simulink model "mpc_cstr_multiple"  (R2025a)
settings: Solver=ode45  StartTime=0  StopTime=60  RelTol=1e-3  EnableMultiTasking=on
values from neighbouring files (symbols this model uses):
  mpcobj = mpc(plant,Ts)    [mpccstr.m]
undefined symbols (not defined in the file or in its folder): CSTR_Setpoints
libraries: mpclib x1
settings Model: Creator=The MathWorks, Inc.  LastModifiedBy=The MathWorks, Inc.
settings SolverCC: AlgebraicLoopSolver=TrustRegion
settings DataIOCC: InitialState=[311.261171037073;8.57000022595505;298.146416805263]  SaveFormat=StructureWithTime  SaveOutput=off  SaveState=on  SignalLogging=off  SaveTime=off  ReturnWorkspaceOutputs=off  SignalLoggingName=logsOut
settings OptimizationCC: BooleanDataType=off  DefaultParameterBehavior=Inlined  InlineInvariantSignals=on  BufferReuse=off  ExpressionDepthLimit=2147483647.0  InitFltsAndDblsToZero=on  EfficientMapNaN2IntZero=off  LifeSpan=inf
settings DebuggingCC: AlgebraicLoopMsg=none  SaveWithParameterizedLinksMsg=none  UnderspecifiedInitializationDetection=Classic  MergeDetectMultiDrivingBlocksExec=none  CheckExecutionContextPreStartOutputMsg=on  SignalResolutionControl=TryResolveAllWithWarning  MultiTaskDSMMsg=warning  MultiTaskCondExecSysMsg=none  FcnCallInpInsideContextMsg=warning  StateNameClashWarn=warning  SFUnexpectedBacktrackingDiag=warning  SFNoUnconditionalDefaultTransitionDiag=warning  SFExecutionAtInitializationDiag=none  ArithmeticOperatorsInVariantConditions=warning
settings HardwareCC: ProdBitPerPointer=32.0  ProdBitPerSizeT=32.0  ProdBitPerPtrDiffT=32.0  ProdLargestAtomicFloat=None  ProdIntDivRoundTo=Undefined  ProdEndianess=Unspecified  ProdWordSize=32.0  ProdHWDeviceType=32-bit Generic  TargetUnknown=on
settings ModelReferenceCC: EnableRefExpFcnMdlSchedulingChecks=on  PropagateSignalLabelsOutOfModel=off
settings SFSimCC: SimUseLocalCustomCode=off  CustomCodeUndefinedFunction=UseInterfaceOnly
settings RTWCC: RTWUseLocalCustomCode=off  GPUComputeCapability=3.5
settings CodeAppCC: StateflowObjectComments=on
settings GRTTargetCC: TargetFcnLib=ansi_tfl_tmw.mat  TargetLangStandard=C89/C90 (ANSI)  CombineOutputUpdateFcns=off  GRTInterface=on
settings ConfigComp: CovMetricSettings=dw  CovSaveCumulativeToWorkspaceVar=on  CovSaveSingleToWorkspaceVar=on  CovExternalEMLEnable=off  CovSFcnEnable=off

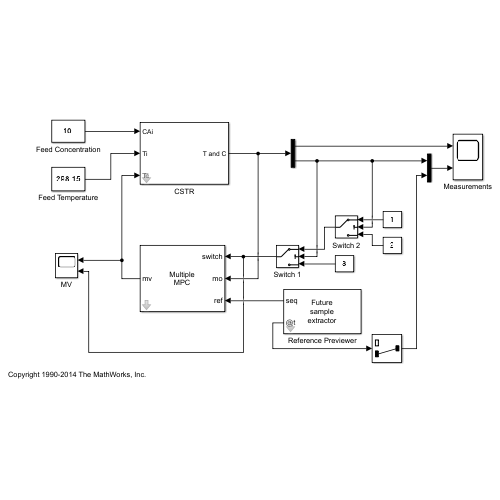
[thumbnail: Simulink's stored preview of the top-level diagram]
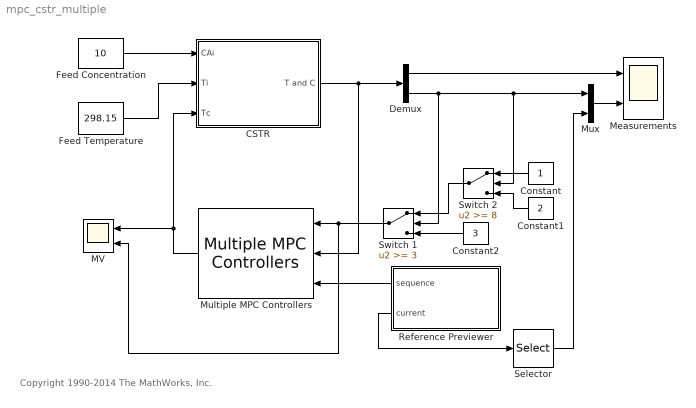
== system mpc_cstr_multiple ==
  note: Copyright 1990-2014 The MathWorks, Inc.
  CSTR : Subsystem  mask{T0=311.2760, C0=8.5695}
      mask prompts: T0 "Initial reactor temperature, K"; C0 "Initial reactor concentration, kmol/m^3"
  Constant : Constant
  Constant1 : Constant  Value=2
  Constant2 : Constant  Value=3
  Demux : Demux  Outputs=2
  Feed Concentration : Constant  Value=10  SampleTime=0
  Feed Temperature : Constant  Value=298.15  SampleTime=0
  MV : Scope  NumInputPorts=2
      settings: TimeSpan=60  Title=Coolant Temperature, K  ActiveDisplayYMinimum=290  ActiveDisplayYMaximum=315
  Measurements : Scope  NumInputPorts=2
      settings: TimeSpan=60  Title=Reactor Temperature, K  ActiveDisplayYMinimum=300  ActiveDisplayYMaximum=380
  Multiple MPC Controllers : mpclib/Multiple MPC Controllers  mpcobjs={'mpcobj','mpcobj_intermediate','mpcobj_final'}  x0s={'[]','[]','[]'}  Nmpc=3  theMPC=3  nmv=1  nmo=0  nmd=0  nts=0  md_inport_multiple=off  mv_inport_multiple=off  uref_inport_multiple=off  return_cost_multiple=off  return_mvseq_multiple=off  return_qpstatus_multiple=off  return_xseq_multiple=off  return_state_multiple=off  return_ovseq_multiple=off  state_inport_multiple=off  umin_inport_multiple=off  umax_inport_multiple=off  ymin_inport_multiple=off  ymax_inport_multiple=off  ywt_inport_multiple=off  uwt_inport_multiple=off  duwt_inport_multiple=off  rhoeps_inport_multiple=off  BlockDataType_multiple=double  SampleTimeInherited_multiple=off
  Mux : Mux  Inputs=2
  Reference Previewer : Subsystem  mask{signal=CSTR_Setpoints, ts=mpcobj.Ts, steps=mpcobj.p}
      mask prompts: signal "Signal name"; ts "Sampling time"; steps "Number of previewing steps"
      mask init:
      | ts = evalin('base',get_param(gcbh,'ts'));
      | signal = evalin('base',get_param(gcbh,'signal'));
      | steps = evalin('base',get_param(gcbh,'steps'));
      | data = mpc_previewer_maskinit(signal,ts);
      mask Display:
      | fprintf('Future\nsample\nextractor');
      | port_label('output', 1, 'seq')
      | port_label('output', 2, '@t')
  Selector : Selector  InputPortWidth=2  IndexOptions=Index vector (dialog)  Indices=2  OutputSizes=1
  Switch 1 : Switch  Threshold=3  SaturateOnIntegerOverflow=off  InputSameDT=off
  Switch 2 : Switch  Threshold=8  SaturateOnIntegerOverflow=off  InputSameDT=off
  wires:
  Feed Concentration/1 -> CSTR/1(CAi)
  Multiple MPC Controllers/1 -> CSTR/3(Tc), MV/1
  Feed Temperature/1 -> CSTR/2(Ti)
  Constant/1 -> Switch 2/1
  Demux/1 -> Measurements/1
  Demux/2 -> Switch 2/2, Mux/1, Switch 1/2
  CSTR/1(T and C) -> Demux/1, Multiple MPC Controllers/2
  Constant1/1 -> Switch 2/3
  Reference Previewer/1(sequence) -> Multiple MPC Controllers/3
  Mux/1 -> Measurements/2
  Selector/1 -> Mux/2
  Switch 1/1 -> MV/2, Multiple MPC Controllers/1
  Constant2/1 -> Switch 1/3
  Switch 2/1 -> Switch 1/1
  Reference Previewer/2(current) -> Selector/1

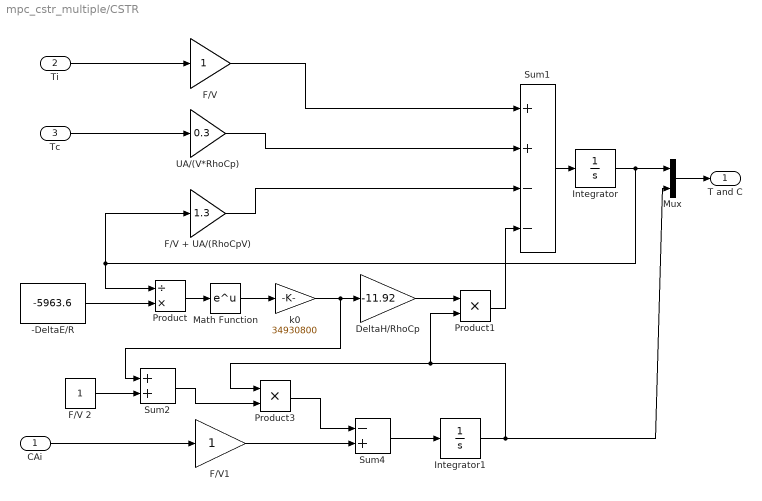
== system mpc_cstr_multiple/CSTR ==
  CAi : Inport
  Ti : Inport  Port=2
  Tc : Inport  Port=3
  -DeltaE/R : Constant  Value=-5963.6  SampleTime=0
  DeltaH/RhoCp : Gain  Gain=-11.92  SaturateOnIntegerOverflow=on  OutDataTypeStr=Inherit: Same as input  ParamDataTypeStr=Inherit: Same as input
  F/V : Gain  SaturateOnIntegerOverflow=on  OutDataTypeStr=Inherit: Same as input  ParamDataTypeStr=Inherit: Same as input
  F/V + UA/(RhoCpV) : Gain  Gain=1.3  SaturateOnIntegerOverflow=on  OutDataTypeStr=Inherit: Same as input  ParamDataTypeStr=Inherit: Same as input
  F/V 2 : Constant  SampleTime=0
  F/V1 : Gain  SaturateOnIntegerOverflow=on  OutDataTypeStr=Inherit: Same as input  ParamDataTypeStr=Inherit: Same as input
  Integrator : Integrator  InitialCondition=311.267  LimitOutput=on  LowerSaturationLimit=0
  Integrator1 : Integrator  InitialCondition=C0  LimitOutput=on  LowerSaturationLimit=0
  Math Function : Math  SignedPower=on
  Mux : Mux  Inputs=2
  Product : Product  Inputs=/*  InputSameDT=on  RndMeth=Zero  SaturateOnIntegerOverflow=on  OutDataTypeStr=Inherit: Same as first input
  Product1 : Product  InputSameDT=on  RndMeth=Zero  SaturateOnIntegerOverflow=on  OutDataTypeStr=Inherit: Same as first input
  Product3 : Product  InputSameDT=on  RndMeth=Zero  SaturateOnIntegerOverflow=on  OutDataTypeStr=Inherit: Same as first input
  Sum1 : Sum  Inputs=++--  InputSameDT=on  SaturateOnIntegerOverflow=on  OutDataTypeStr=Inherit: Same as first input
  Sum2 : Sum  InputSameDT=on  SaturateOnIntegerOverflow=on  OutDataTypeStr=Inherit: Same as first input
  Sum4 : Sum  Inputs=-+  InputSameDT=on  SaturateOnIntegerOverflow=on  OutDataTypeStr=Inherit: Same as first input
  UA/(V*RhoCp) : Gain  Gain=0.3  SaturateOnIntegerOverflow=on  OutDataTypeStr=Inherit: Same as input  ParamDataTypeStr=Inherit: Same as input
  k0 : Gain  Gain=34930800  SaturateOnIntegerOverflow=on  OutDataTypeStr=Inherit: Same as input  ParamDataTypeStr=Inherit: Same as input
  T and C : Outport
  wires:
  F/V/1 -> Sum1/1
  Sum1/1 -> Integrator/1
  Integrator/1 -> Product/1, F/V + UA/(RhoCpV)/1, Mux/1
  UA/(V*RhoCp)/1 -> Sum1/2
  F/V + UA/(RhoCpV)/1 -> Sum1/3
  Product/1 -> Math Function/1
  Math Function/1 -> k0/1
  DeltaH/RhoCp/1 -> Product1/1
  Product1/1 -> Sum1/4
  k0/1 -> DeltaH/RhoCp/1, Sum2/1
  -DeltaE/R/1 -> Product/2
  Product3/1 -> Sum4/1
  Sum4/1 -> Integrator1/1
  Integrator1/1 -> Product3/1, Product1/2, Mux/2
  F/V 2/1 -> Sum2/2
  F/V1/1 -> Sum4/2
  Ti/1 -> F/V/1
  CAi/1 -> F/V1/1
  Tc/1 -> UA/(V*RhoCp)/1
  Sum2/1 -> Product3/2
  Mux/1 -> T and C/1

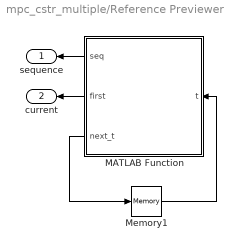
== system mpc_cstr_multiple/Reference Previewer ==
  MATLAB Function : MATLAB Function  TreatAsAtomicUnit=on
  Memory1 : Memory  InheritSampleTime=on  LinearizeAsDelay=on
  sequence : Outport
  current : Outport  Port=2
  wires:
  MATLAB Function/3(next_t) -> Memory1/1
  Memory1/1 -> MATLAB Function/1(t)
  MATLAB Function/2(first) -> current/1
  MATLAB Function/1(seq) -> sequence/1

== matlab function mpc_cstr_multiple/Reference Previewer/MATLAB Function ==
  settings: updateMethod=DISCRETE  sampleTime=ts
  data: data parameter; seq output; steps parameter; t input; first output; next_t output
function [seq,first,next_t] = fcn(data,steps,t)
%#codegen
[seq,first,next_t] = mpcblock_preview('ref',data,steps,t);
